simulink model "LTS_testing"  (R2025b)
settings: Solver=ode23t  StartTime=0.0  StopTime=1
model workspace: external: MATLAB File C:\Users\thoma\Documents\ME-Steering-2026\MATLAB\VD\LTS.m (data not in the file)
undefined symbols (not defined in the file): AR26
libraries: vehdynlibtire x4, autolibshared x2, vehdynlibdriver x1, simulink x1, autolibmappedmotor x1, autolibsharedcoupling x1, vehdynlibsteering x1
(part 2 of 2)

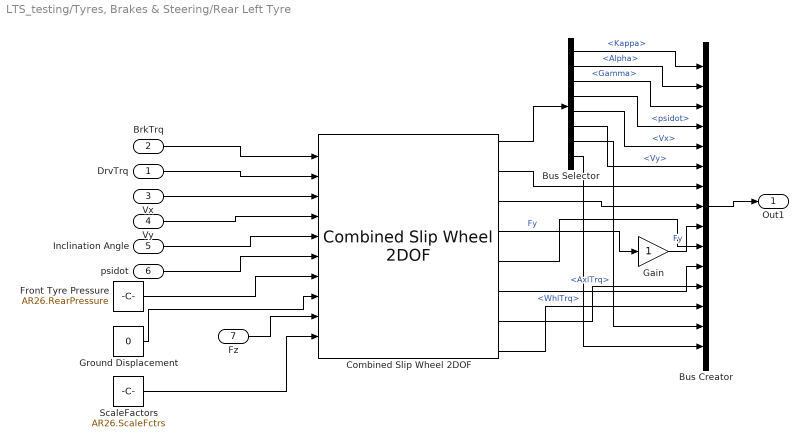
== system LTS_testing/Tyres, Brakes & Steering/Rear Left Tyre ==
  DrvTrq : Inport
  BrkTrq : Inport  Port=2
  Vx : Inport  Port=3
  Vy : Inport  Port=4
  Inclination Angle : Inport  Port=5
  psidot : Inport  Port=6
  Fz : Inport  Port=7
  Bus Creator : BusCreator  Inputs=15
  Bus Selector : BusSelector  OutputSignals=Kappa,Alpha,Gamma,psidot,Vx,Vy,AxlTrq,WhlTrq
  Combined Slip Wheel 2DOF : vehdynlibtire/Combined Slip Wheel 2DOF  tireType=External file  tireParamSet=C:\Users\thoma\Documents\ME-Steering-2026\MATLAB\VD\left.tir  vertType=Magic Formula  plySteer=off  turnslip=off  BrakeType=Disc  mu_static=.3  mu_kinetic=.2  drum_abore=0.0508  drum_a=0.123  drum_c=0.212  drum_r=0.15  drum_theta1=0  drum_theta2=126  disk_abore=AR26.PistonDiam  Rm=AR26.DiscRadius  num_pads=AR26.NPistonAxle  brake_p_bpt=[1 11.4736842105263 21.9473684210526 32.4210526315789 42.8947368421053 53.3684210526316 63.8421052631579 74.3157894736842 84.7894736842105 95.2631578947368 105.736842105263 116.210526315789 126.684210526316 137.157894736842 147.631578947368 158.105263157895 168.578947368421 179.052631578947 189.526315789474 200]  brake_n_bpt=[0 52.6315789473684 105.263157894737 157.894736842105 210.526315789474 263.157894736842 315.789473684211 368.421052631579 421.052631578947 473.684210526316 526.315789473684 578.947368421053 631.578947368421 684.210526315789 736.842105263158 789.473684210526 842.105263157895 894.736842105263 947.368421052632 1000]  f_brake_t=[43.4900602404453 42.5056030554862 41.5350898940194 40.5780454442085 39.6340111501808 38.7025443887544 37.7832176914519 36.8756180088306 35.9793460143796 35.0940154454303 34.2192524787115 33.3546951383474 32.4999927342521 31.6548053290159 30.8188032315107 29.991666515561 29.1730845621415 28.362755623661 27.5603864089927 26.765691687993;498.991217495636 487.695866636631 476.560505099801 465.579679307235 454.748127933653 444.060772460445 433.51270824929 423.099196101319 412.81565427025 402.657650900201 392.620896861006 382.701238955775 372.894653477208 363.197240090814 353.605216024701 344.114910546964 334.722759712992 325.425301366216 316.219170376863 307.10109410434;954.492374750826 932.886130217776 911.585920305583 890.581313170261 869.862244717126 849.419000532136 829.242198807128 809.322774193808 789.651962526121 770.221286354971 751.0225412433 732.047782773203 713.289314220164 694.739674852612 676.391628817892 658.238154578366 640.272434863842 622.48784710877 604.877954344734 587.436496520688;1409.99353200602 1378.07639379892 1346.61133551136 1315.58294703329 1284.9763615006 1254.77722860383 1224.97168936497 1195.5463522863 1166.48827078199 1137.78492180974 1109.42418562559 1081.39432659063 1053.68397496312 1026.28210961441 999.178041611083 972.361398609768 945.822110014692 919.550392851325 893.536738312604 867.771898937035;1865.49468926121 1823.26665738007 1781.63675071715 1740.58458089631 1700.09047828407 1660.13545667552 1620.7011799228 1581.76993037878 1543.32457903786 1505.34855726451 1467.82583000789 1430.74087040806 1394.07863570608 1357.82454437621 1321.96445440427 1286.48464264117 1251.37178516554 1216.61293859388 1182.19552228048 1148.10730135338;2320.9958465164 2268.45692096121 2216.66216592293 2165.58621475934 2115.20459506754 2065.49368474721 2016.43067048064 1967.99350847127 1920.16088729373 1872.91219271928 1826.22747439018 1780.08741422549 1734.47329644903 1689.36697913801 1644.75086719747 1600.60788667257 1556.92146031639 1513.67548433643 1470.85430624835 1428.44270376973;2776.49700377159 2713.64718454235 2651.68758112871 2590.58784862237 2530.31871185102 2470.8519128189 2412.16016103848 2354.21708656376 2296.9971955496 2240.47582817405 2184.62911877248 2129.43395804292 2074.86795719199 2020.9094138998 1967.53727999066 1914.73113070398 1862.47113546724 1810.73803007899 1759.51309021622 1708.77810618608;3231.99816102678 3158.8374481235 3086.71299633449 3015.58948248539 2945.43282863449 2876.21014089059 2807.88965159632 2740.44066465625 2673.83350380547 2608.03946362882 2543.03076315477 2478.78050186034 2415.26261793494 2352.4518486616 2290.32369278385 2228.85437473538 2168.02081061809 2107.80057582154 2048.17187418409 1989.11350860242;3687.49931828197 3604.02771170464 3521.73841154027 3440.59111634842 3360.54694541796 3281.56836896228 3203.61914215416 3126.66424274874 3050.66981206134 2975.60309908359 2901.43240753707 2828.12704567777 2755.6572786779 2683.9942834234 2613.11010557704 2542.97761876678 2473.57048576894 2404.8631215641 2336.83065815196 2269.44891101877;4143.00047553716 4049.21797528579 3956.76382674606 3865.59275021144 3775.66106220143 3686.92659703397 3599.34863271199 3512.88782084123 3427.50612031721 3343.16673453836 3259.83405191936 3177.4735894952 3096.05193942085 3015.5367181852 2935.89651837023 2857.10086279818 2779.12016091979 2701.92566730665 2625.48944211983 2549.78431343512;4598.50163279235 4494.40823886693 4391.78924195184 4290.59438407447 4190.77517898491 4092.28482510566 3995.07812326983 3899.11139893372 3804.34242857308 3710.73036999313 3618.23569630166 3526.82013331263 3436.44660016381 3347.079152947 3258.68293116342 3171.22410682959 3084.66983607064 2998.98821304921 2914.1482260877 2830.11971585147;5054.00279004754 4939.59850244808 4826.81465715762 4715.59601793749 4605.88929576838 4497.64305317735 4390.80761382767 4285.3349770262 4181.17873682896 4078.2940054479 3976.63734068395 3876.16667713006 3776.84126090677 3678.62158770879 3581.46934395661 3485.34735086099 ...(+2764 chars)]  NOMPRES=84000  PRESMAX=1000000  PRESMIN=10000  FNOMIN=750  FZMAX=8600  FZMIN=100  VXLOW=0.01  KPUMAX=AR26.KappaMax  KPUMIN=AR26.KappaMin  ALPMAX=1.5  ALPMIN=-1.5  CAMMAX=0.17453  CAMMIN=-0.17453  LONGVL=25  FxRelFreqLwrLim=200*pi  FyRelFreqLwrLim=200*pi  MyRelFreqLwrLim=100*pi  omegao=AR26.Omega0  UNLOADED_RADIUS=0.203  WIDTH=AR26.TireWidth  RIM_RADIUS=AR26.RimRadius  ASPECT_RATIO=0.45  MASS=11.2  IYY=1.084  br=1e-3  GRAVITY=-9.81  zo=0  zdoto=0  BREFF=8.25094594147963  DREFF=0.260468730454265  FREFF=0.0735298544471851  Q_RE0=1.00866439868088  Q_V1=0.000760413786224011  Q_V2=0.0463384792019201  Q_FZ1=0  Q_FZ2=15.6870832810226  Q_FZ3=0  Q_FCX=0.138643970247602  Q_FCY=0.10843499565426  Q_FCY2=-0.465763352339538  PFZ1=0.69958166705601  VERTICAL_STIFFNESS=207885.061134007  VERTICAL_DAMPING=500  BOTTOM_OFFST=0.00990653336182505  BOTTOM_STIFF=1999075.87051971  Q_CAM1=86.7791723017291  Q_CAM2=259.705254231766  Q_CAM3=0.510281667378416  Q_FYS1=-20769.4728880343  Q_FYS2=-59060.183485617  Q_FYS3=89271.8260126986  LONGITUDINAL_STIFFNESS=388714.175879854  LATERAL_STIFFNESS=157087.404633332  PCFX1=0.18539229191199  PCFX2=0  PCFX3=0  PCFY1=0.163183345037677  PCFY2=0  PCFY3=0.249094918231954  Q_RA1=0.675942571700787  Q_RA2=0.73800463546164  Q_RB1=1.04487486456705  Q_RB2=-1.191763806629  PCX1=1.5  PDX1=2.5435  PDX2=-0.64632  PDX3=11.0199  PEX1=-6.4596e-11  PEX2=-0.84982  PEX3=-0.6  PEX4=0.9  PKX1=42.6771  PKX2=-0.011985  PKX3=-0.53674  PHX1=0.0017597  PHX2=-0.001133  PVX1=-0.085025  PVX2=0.1  PPX1=0.25355  PPX2=12.2145  PPX3=-0.055934  PPX4=-2.6628  RBX1=5  RBX2=5  RBX3=0  RCX1=1  REX1=-1  REX2=-0.1  RHX1=0  QSX1=0  QSX2=1.5  QSX3=0.1  QSX4=0.1  QSX5=0  QSX6=0  QSX7=0.1  QSX8=0  QSX9=0  QSX10=0  QSX11=0  QSX12=0  QSX13=0  QSX14=0  PPMX1=0  PCY1=1.5  PDY1=2.1471  PDY2=-0.42791  PDY3=8.3327  PEY1=0.35224  PEY2=-0.17141  PEY3=0.10605  PEY4=-3.7833  PEY5=-62.9571  PKY1=-31.419  PKY2=1.5115  PKY3=0.30996  PKY4=2  PKY5=38.0826  PKY6=-3.9753  PKY7=-1.8011  PHY1=0.0024113  PHY2=0.00049845  PVY1=0.10412  PVY2=-0.053643  PVY3=0.53589  PVY4=1.2244  PPY1=0.40814  PPY2=1.0811  PPY3=-0.51005  PPY4=-0.29281  PPY5=-0.8874  RBY1=5  RBY2=2  RBY3=0.02  RBY4=0  RCY1=1  REY1=-0.1  REY2=0.1  RHY1=0  RHY2=0  RVY1=0  RVY2=0  RVY3=0  RVY4=0  RVY5=0  RVY6=0  QSY1=0  QSY2=0  QSY3=0  QSY4=0  QSY5=0  QSY6=0  QSY7=0  QSY8=0  QBZ1=0.36866  QBZ2=0.87296  QBZ3=0.64959  QBZ4=168.8149  QBZ5=-172.3075  QBZ6=0  QBZ9=-33.2482  QBZ10=-2.3968  QCZ1=14.2367  QDZ1=0.10605  QDZ2=-0.11593  QDZ3=4.9221  QDZ4=-8.2609  QDZ6=-0.023114  QDZ7=0.034508  QDZ8=-0.92786  QDZ9=2.4605  QDZ10=-11.696  QDZ11=-63.4068  QEZ1=-0.069508  QEZ2=-0.3322  QEZ3=-0.2814  QEZ4=3.6678  QEZ5=-275.1131  QHZ1=-0.019925  QHZ2=1.2787  QHZ3=-1.7534  QHZ4=0.77276  PPZ1=0  PPZ2=0  SSZ1=0  SSZ2=0  SSZ3=0  SSZ4=0  PDXP1=0  PDXP2=0  PDXP3=0  PKYP1=0  PDYP1=0  PDYP2=0  PDYP3=0  PDYP4=0  PHYP1=0  PHYP2=0  PHYP3=0  PHYP4=0  PECP1=0  PECP2=0  QDTP1=0  QCRP1=0  QCRP2=0  QBRP1=0  QDRP1=0  QDRP2=0  aMode=2
  Front Tyre Pressure : Constant  Value=AR26.RearPressure
  Gain : Gain
  Ground Displacement : Constant  Value=0
  ScaleFactors : Constant  Value=AR26.ScaleFctrs
  Out1 : Outport
  wires:
  Vy/1 -> Combined Slip Wheel 2DOF/4
  Ground Displacement/1 -> Combined Slip Wheel 2DOF/8
  Combined Slip Wheel 2DOF/3 -> Bus Creator/8
  Inclination Angle/1 -> Combined Slip Wheel 2DOF/5
  DrvTrq/1 -> Combined Slip Wheel 2DOF/2
  Bus Creator/1 -> Out1/1
  BrkTrq/1 -> Combined Slip Wheel 2DOF/1
  Combined Slip Wheel 2DOF/8 -> Bus Creator/13
  psidot/1 -> Combined Slip Wheel 2DOF/6
  Front Tyre Pressure/1 -> Combined Slip Wheel 2DOF/7
  Combined Slip Wheel 2DOF/2 -> Bus Creator/7
  Combined Slip Wheel 2DOF/6 -> Bus Creator/11
  Combined Slip Wheel 2DOF/5 -> Bus Creator/10
  Combined Slip Wheel 2DOF/7 -> Bus Creator/12
  ScaleFactors/1 -> Combined Slip Wheel 2DOF/10
  Fz/1 -> Combined Slip Wheel 2DOF/9
  Vx/1 -> Combined Slip Wheel 2DOF/3
  Bus Selector/5 -> Bus Creator/5  "<Vx>"
  Bus Selector/6 -> Bus Creator/6  "<Vy>"
  Combined Slip Wheel 2DOF/1 -> Bus Selector/1
  Bus Selector/1 -> Bus Creator/1  "<Kappa>"
  Bus Selector/2 -> Bus Creator/2  "<Alpha>"
  Bus Selector/3 -> Bus Creator/3  "<Gamma>"
  Bus Selector/4 -> Bus Creator/4  "<psidot>"
  Combined Slip Wheel 2DOF/4 -> Gain/1  "Fy"
  Gain/1 -> Bus Creator/9  "Fy"
  Bus Selector/8 -> Bus Creator/15  "<WhlTrq>"
  Bus Selector/7 -> Bus Creator/14  "<AxlTrq>"

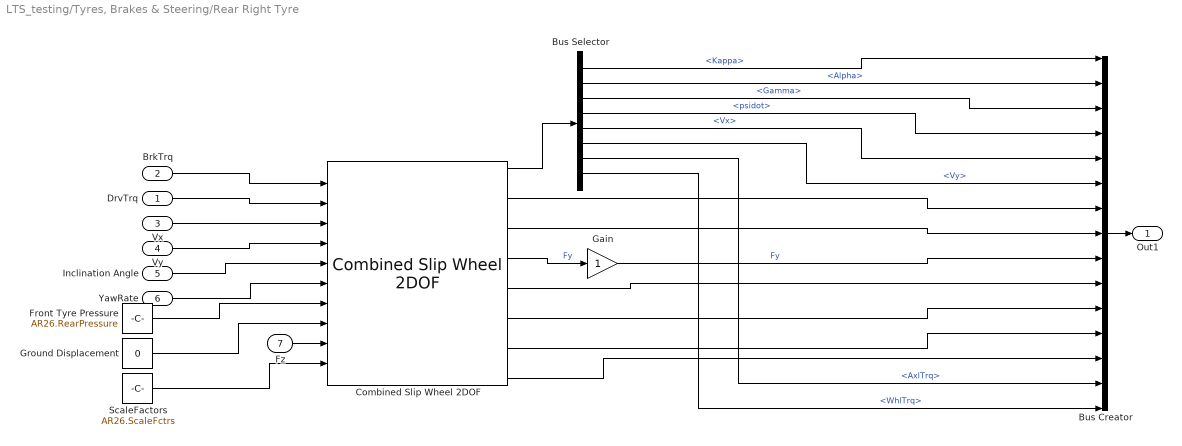
== system LTS_testing/Tyres, Brakes & Steering/Rear Right Tyre ==
  DrvTrq : Inport
  BrkTrq : Inport  Port=2
  Vx : Inport  Port=3
  Vy : Inport  Port=4
  Inclination Angle : Inport  Port=5
  YawRate : Inport  Port=6
  Fz : Inport  Port=7
  Bus Creator : BusCreator  Inputs=15
  Bus Selector : BusSelector  OutputSignals=Kappa,Alpha,Gamma,psidot,Vx,Vy,AxlTrq,WhlTrq
  Combined Slip Wheel 2DOF : vehdynlibtire/Combined Slip Wheel 2DOF  tireType=External file  tireParamSet=C:\Users\thoma\Documents\ME-Steering-2026\MATLAB\VD\right.tir  vertType=Magic Formula  plySteer=off  turnslip=off  BrakeType=Disc  mu_static=.3  mu_kinetic=.2  drum_abore=0.0508  drum_a=0.123  drum_c=0.212  drum_r=0.15  drum_theta1=0  drum_theta2=126  disk_abore=AR26.PistonDiam  Rm=AR26.DiscRadius  num_pads=AR26.NPistonAxle  brake_p_bpt=[1 11.4736842105263 21.9473684210526 32.4210526315789 42.8947368421053 53.3684210526316 63.8421052631579 74.3157894736842 84.7894736842105 95.2631578947368 105.736842105263 116.210526315789 126.684210526316 137.157894736842 147.631578947368 158.105263157895 168.578947368421 179.052631578947 189.526315789474 200]  brake_n_bpt=[0 52.6315789473684 105.263157894737 157.894736842105 210.526315789474 263.157894736842 315.789473684211 368.421052631579 421.052631578947 473.684210526316 526.315789473684 578.947368421053 631.578947368421 684.210526315789 736.842105263158 789.473684210526 842.105263157895 894.736842105263 947.368421052632 1000]  f_brake_t=[43.4900602404453 42.5056030554862 41.5350898940194 40.5780454442085 39.6340111501808 38.7025443887544 37.7832176914519 36.8756180088306 35.9793460143796 35.0940154454303 34.2192524787115 33.3546951383474 32.4999927342521 31.6548053290159 30.8188032315107 29.991666515561 29.1730845621415 28.362755623661 27.5603864089927 26.765691687993;498.991217495636 487.695866636631 476.560505099801 465.579679307235 454.748127933653 444.060772460445 433.51270824929 423.099196101319 412.81565427025 402.657650900201 392.620896861006 382.701238955775 372.894653477208 363.197240090814 353.605216024701 344.114910546964 334.722759712992 325.425301366216 316.219170376863 307.10109410434;954.492374750826 932.886130217776 911.585920305583 890.581313170261 869.862244717126 849.419000532136 829.242198807128 809.322774193808 789.651962526121 770.221286354971 751.0225412433 732.047782773203 713.289314220164 694.739674852612 676.391628817892 658.238154578366 640.272434863842 622.48784710877 604.877954344734 587.436496520688;1409.99353200602 1378.07639379892 1346.61133551136 1315.58294703329 1284.9763615006 1254.77722860383 1224.97168936497 1195.5463522863 1166.48827078199 1137.78492180974 1109.42418562559 1081.39432659063 1053.68397496312 1026.28210961441 999.178041611083 972.361398609768 945.822110014692 919.550392851325 893.536738312604 867.771898937035;1865.49468926121 1823.26665738007 1781.63675071715 1740.58458089631 1700.09047828407 1660.13545667552 1620.7011799228 1581.76993037878 1543.32457903786 1505.34855726451 1467.82583000789 1430.74087040806 1394.07863570608 1357.82454437621 1321.96445440427 1286.48464264117 1251.37178516554 1216.61293859388 1182.19552228048 1148.10730135338;2320.9958465164 2268.45692096121 2216.66216592293 2165.58621475934 2115.20459506754 2065.49368474721 2016.43067048064 1967.99350847127 1920.16088729373 1872.91219271928 1826.22747439018 1780.08741422549 1734.47329644903 1689.36697913801 1644.75086719747 1600.60788667257 1556.92146031639 1513.67548433643 1470.85430624835 1428.44270376973;2776.49700377159 2713.64718454235 2651.68758112871 2590.58784862237 2530.31871185102 2470.8519128189 2412.16016103848 2354.21708656376 2296.9971955496 2240.47582817405 2184.62911877248 2129.43395804292 2074.86795719199 2020.9094138998 1967.53727999066 1914.73113070398 1862.47113546724 1810.73803007899 1759.51309021622 1708.77810618608;3231.99816102678 3158.8374481235 3086.71299633449 3015.58948248539 2945.43282863449 2876.21014089059 2807.88965159632 2740.44066465625 2673.83350380547 2608.03946362882 2543.03076315477 2478.78050186034 2415.26261793494 2352.4518486616 2290.32369278385 2228.85437473538 2168.02081061809 2107.80057582154 2048.17187418409 1989.11350860242;3687.49931828197 3604.02771170464 3521.73841154027 3440.59111634842 3360.54694541796 3281.56836896228 3203.61914215416 3126.66424274874 3050.66981206134 2975.60309908359 2901.43240753707 2828.12704567777 2755.6572786779 2683.9942834234 2613.11010557704 2542.97761876678 2473.57048576894 2404.8631215641 2336.83065815196 2269.44891101877;4143.00047553716 4049.21797528579 3956.76382674606 3865.59275021144 3775.66106220143 3686.92659703397 3599.34863271199 3512.88782084123 3427.50612031721 3343.16673453836 3259.83405191936 3177.4735894952 3096.05193942085 3015.5367181852 2935.89651837023 2857.10086279818 2779.12016091979 2701.92566730665 2625.48944211983 2549.78431343512;4598.50163279235 4494.40823886693 4391.78924195184 4290.59438407447 4190.77517898491 4092.28482510566 3995.07812326983 3899.11139893372 3804.34242857308 3710.73036999313 3618.23569630166 3526.82013331263 3436.44660016381 3347.079152947 3258.68293116342 3171.22410682959 3084.66983607064 2998.98821304921 2914.1482260877 2830.11971585147;5054.00279004754 4939.59850244808 4826.81465715762 4715.59601793749 4605.88929576838 4497.64305317735 4390.80761382767 4285.3349770262 4181.17873682896 4078.2940054479 3976.63734068395 3876.16667713006 3776.84126090677 3678.62158770879 3581.46934395661 3485.34735086099 ...(+2764 chars)]  NOMPRES=84000  PRESMAX=1000000  PRESMIN=10000  FNOMIN=750  FZMAX=8600  FZMIN=100  VXLOW=0.01  KPUMAX=AR26.KappaMax  KPUMIN=AR26.KappaMin  ALPMAX=1.5  ALPMIN=-1.5  CAMMAX=0.17453  CAMMIN=-0.17453  LONGVL=25  FxRelFreqLwrLim=200*pi  FyRelFreqLwrLim=200*pi  MyRelFreqLwrLim=100*pi  omegao=AR26.Omega0  UNLOADED_RADIUS=0.203  WIDTH=AR26.TireWidth  RIM_RADIUS=AR26.RimRadius  ASPECT_RATIO=0.45  MASS=11.2  IYY=1.084  br=1e-3  GRAVITY=-9.81  zo=0  zdoto=0  BREFF=8.25094594147963  DREFF=0.260468730454265  FREFF=0.0735298544471851  Q_RE0=1.00866439868088  Q_V1=0.000760413786224011  Q_V2=0.0463384792019201  Q_FZ1=0  Q_FZ2=15.6870832810226  Q_FZ3=0  Q_FCX=0.138643970247602  Q_FCY=0.10843499565426  Q_FCY2=-0.465763352339538  PFZ1=0.69958166705601  VERTICAL_STIFFNESS=207885.061134007  VERTICAL_DAMPING=500  BOTTOM_OFFST=0.00990653336182505  BOTTOM_STIFF=1999075.87051971  Q_CAM1=86.7791723017291  Q_CAM2=259.705254231766  Q_CAM3=0.510281667378416  Q_FYS1=-20769.4728880343  Q_FYS2=-59060.183485617  Q_FYS3=89271.8260126986  LONGITUDINAL_STIFFNESS=388714.175879854  LATERAL_STIFFNESS=157087.404633332  PCFX1=0.18539229191199  PCFX2=0  PCFX3=0  PCFY1=0.163183345037677  PCFY2=0  PCFY3=0.249094918231954  Q_RA1=0.675942571700787  Q_RA2=0.73800463546164  Q_RB1=1.04487486456705  Q_RB2=-1.191763806629  PCX1=1.5  PDX1=2.5435  PDX2=-0.64632  PDX3=11.0199  PEX1=-6.4596e-11  PEX2=-0.84982  PEX3=-0.6  PEX4=0.9  PKX1=42.6771  PKX2=-0.011985  PKX3=-0.53674  PHX1=0.0017597  PHX2=-0.001133  PVX1=-0.085025  PVX2=0.1  PPX1=0.25355  PPX2=12.2145  PPX3=-0.055934  PPX4=-2.6628  RBX1=5  RBX2=5  RBX3=0  RCX1=1  REX1=-1  REX2=-0.1  RHX1=0  QSX1=0  QSX2=1.5  QSX3=0.1  QSX4=0.1  QSX5=0  QSX6=0  QSX7=0.1  QSX8=0  QSX9=0  QSX10=0  QSX11=0  QSX12=0  QSX13=0  QSX14=0  PPMX1=0  PCY1=1.5  PDY1=2.1471  PDY2=-0.42791  PDY3=8.3327  PEY1=0.35224  PEY2=-0.17141  PEY3=0.10605  PEY4=-3.7833  PEY5=-62.9571  PKY1=-31.419  PKY2=1.5115  PKY3=0.30996  PKY4=2  PKY5=38.0826  PKY6=-3.9753  PKY7=-1.8011  PHY1=0.0024113  PHY2=0.00049845  PVY1=0.10412  PVY2=-0.053643  PVY3=0.53589  PVY4=1.2244  PPY1=0.40814  PPY2=1.0811  PPY3=-0.51005  PPY4=-0.29281  PPY5=-0.8874  RBY1=5  RBY2=2  RBY3=0.02  RBY4=0  RCY1=1  REY1=-0.1  REY2=0.1  RHY1=0  RHY2=0  RVY1=0  RVY2=0  RVY3=0  RVY4=0  RVY5=0  RVY6=0  QSY1=0  QSY2=0  QSY3=0  QSY4=0  QSY5=0  QSY6=0  QSY7=0  QSY8=0  QBZ1=0.36866  QBZ2=0.87296  QBZ3=0.64959  QBZ4=168.8149  QBZ5=-172.3075  QBZ6=0  QBZ9=-33.2482  QBZ10=-2.3968  QCZ1=14.2367  QDZ1=0.10605  QDZ2=-0.11593  QDZ3=4.9221  QDZ4=-8.2609  QDZ6=-0.023114  QDZ7=0.034508  QDZ8=-0.92786  QDZ9=2.4605  QDZ10=-11.696  QDZ11=-63.4068  QEZ1=-0.069508  QEZ2=-0.3322  QEZ3=-0.2814  QEZ4=3.6678  QEZ5=-275.1131  QHZ1=-0.019925  QHZ2=1.2787  QHZ3=-1.7534  QHZ4=0.77276  PPZ1=0  PPZ2=0  SSZ1=0  SSZ2=0  SSZ3=0  SSZ4=0  PDXP1=0  PDXP2=0  PDXP3=0  PKYP1=0  PDYP1=0  PDYP2=0  PDYP3=0  PDYP4=0  PHYP1=0  PHYP2=0  PHYP3=0  PHYP4=0  PECP1=0  PECP2=0  QDTP1=0  QCRP1=0  QCRP2=0  QBRP1=0  QDRP1=0  QDRP2=0  aMode=2
  Front Tyre Pressure : Constant  Value=AR26.RearPressure
  Gain : Gain
  Ground Displacement : Constant  Value=0
  ScaleFactors : Constant  Value=AR26.ScaleFctrs
  Out1 : Outport
  wires:
  ScaleFactors/1 -> Combined Slip Wheel 2DOF/10
  Combined Slip Wheel 2DOF/2 -> Bus Creator/7
  Bus Creator/1 -> Out1/1
  Front Tyre Pressure/1 -> Combined Slip Wheel 2DOF/7
  YawRate/1 -> Combined Slip Wheel 2DOF/6
  Combined Slip Wheel 2DOF/6 -> Bus Creator/11
  Combined Slip Wheel 2DOF/5 -> Bus Creator/10
  Fz/1 -> Combined Slip Wheel 2DOF/9
  Vx/1 -> Combined Slip Wheel 2DOF/3
  Inclination Angle/1 -> Combined Slip Wheel 2DOF/5
  Ground Displacement/1 -> Combined Slip Wheel 2DOF/8
  BrkTrq/1 -> Combined Slip Wheel 2DOF/1
  Combined Slip Wheel 2DOF/7 -> Bus Creator/12
  Combined Slip Wheel 2DOF/8 -> Bus Creator/13
  Vy/1 -> Combined Slip Wheel 2DOF/4
  Combined Slip Wheel 2DOF/3 -> Bus Creator/8
  DrvTrq/1 -> Combined Slip Wheel 2DOF/2
  Bus Selector/5 -> Bus Creator/5  "<Vx>"
  Bus Selector/6 -> Bus Creator/6  "<Vy>"
  Combined Slip Wheel 2DOF/1 -> Bus Selector/1
  Bus Selector/1 -> Bus Creator/1  "<Kappa>"
  Bus Selector/2 -> Bus Creator/2  "<Alpha>"
  Bus Selector/3 -> Bus Creator/3  "<Gamma>"
  Bus Selector/4 -> Bus Creator/4  "<psidot>"
  Combined Slip Wheel 2DOF/4 -> Gain/1  "Fy"
  Gain/1 -> Bus Creator/9  "Fy"
  Bus Selector/8 -> Bus Creator/15  "<WhlTrq>"
  Bus Selector/7 -> Bus Creator/14  "<AxlTrq>"

== system LTS_testing/Tyres, Brakes & Steering/Steering ==
  In1 : Inport
  Bus Selector : BusSelector  OutputSignals=InstStrgRatio
  Kinematic Steering1 : vehdynlibsteering/Kinematic Steering  StrgType=Rack and pinion  StrgRatioType=Lookup table  Loc=Front  NrmlFctr=3  TrckWdth=AR26.FrontTrackwidth  WhlBase=1.524  Db=0  StrgRng=pi  StrgAngBpts=AR26.WheelBreakPoints  StrgRatioTbl=|  StrgRatio=100  PctAckIn=off  PctAck=100  PctAckTbl=ones(1,11)*100  StrgArmLngth=AR26.SteeringArmLength  RckCsLngth=AR26.RackWidth  TieRodLngth=AR26.TieRodLength  D=AR26.RackAxisLength  PnnRadius=AR26.PinionRadius  PnnRadiusTbl=AR26.PinionRadiusTable  RodLngth=0.1  ParaArmLngth=0.9  aMode=2
      | [13.5000   13.3750   13.2500   13.1250   13.0000   13.0000   13.0000   13.1250   13.2500   13.3750   13.5000
      | ]
  Saturation1 : Saturate  UpperLimit=0.61  LowerLimit=-0.61
  Out1 : Outport
  Out2 : Outport  Port=2
  wires:
  Kinematic Steering1/3 -> Out2/1  "FRWheelAngle"
  Kinematic Steering1/2 -> Out1/1  "FLWheelAngle"
  Kinematic Steering1/1 -> Bus Selector/1
  In1/1 -> Kinematic Steering1/1  "SteerIn"

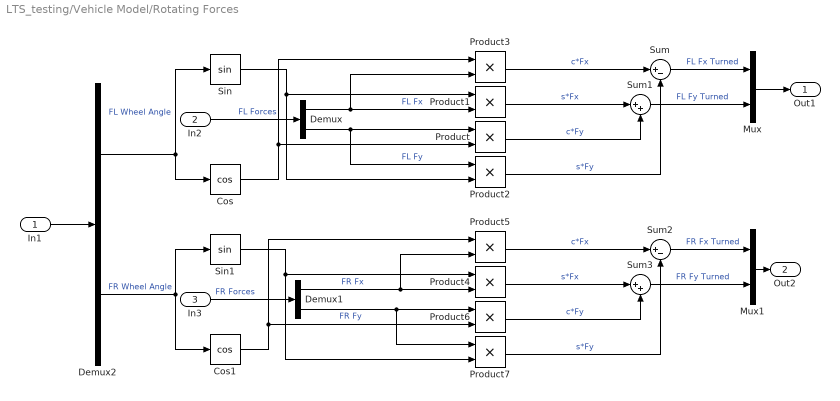
== system LTS_testing/Vehicle Model/Rotating Forces ==
  In1 : Inport
  In2 : Inport  Port=2
  In3 : Inport  Port=3
  Cos : Trigonometry  Operator=cos
  Cos1 : Trigonometry  Operator=cos
  Demux : Demux  Outputs=2
  Demux1 : Demux  Outputs=2
  Demux2 : Demux  Outputs=2
  Mux : Mux  Inputs=2
  Mux1 : Mux  Inputs=2
  Product{,1..7} (8 alike) : Product
  Sin : Trigonometry
  Sin1 : Trigonometry
  Sum : Sum  Inputs=|+-
  Sum1 : Sum  Inputs=|++
  Sum2 : Sum  Inputs=|+-
  Sum3 : Sum  Inputs=|++
  Out1 : Outport
  Out2 : Outport  Port=2
  wires:
  Demux2/2 -> Sin1/1, Cos1/1  "FR Wheel Angle"
  Demux2/1 -> Sin/1, Cos/1  "FL Wheel Angle"
  In1/1 -> Demux2/1
  In2/1 -> Demux/1  "FL Forces"
  Demux/1 -> Product3/2, Product1/2  "FL Fx"
  Demux/2 -> Product2/1, Product/1  "FL Fy"
  Cos/1 -> Product3/1, Product/2
  Product/1 -> Sum1/2  "c*Fy"
  Sin/1 -> Product2/2, Product1/1
  Product1/1 -> Sum1/1  "s*Fx"
  Product2/1 -> Sum/2  "s*Fy"
  Product3/1 -> Sum/1  "c*Fx"
  Sum/1 -> Mux/1  "FL Fx Turned"
  Sum1/1 -> Mux/2  "FL Fy Turned"
  Mux/1 -> Out1/1
  In3/1 -> Demux1/1  "FR Forces"
  Demux1/1 -> Product5/2, Product4/2  "FR Fx"
  Demux1/2 -> Product7/1, Product6/1  "FR Fy"
  Product4/1 -> Sum3/1  "s*Fx"
  Sin1/1 -> Product7/2, Product4/1
  Product5/1 -> Sum2/1  "c*Fx"
  Product6/1 -> Sum3/2  "c*Fy"
  Product7/1 -> Sum2/2  "s*Fy"
  Cos1/1 -> Product5/1, Product6/2
  Sum2/1 -> Mux1/1  "FR Fx Turned"
  Sum3/1 -> Mux1/2  "FR Fy Turned"
  Mux1/1 -> Out2/1
